simulink model "halogen"  (R2018a)
settings: Solver=ode1  StartTime=0.0  StopTime=11  FixedStep=0.1  RelTol=1e-3
values from neighbouring files (symbols this model uses):
  b = [1/6, 1/3, 1/3, 1/6]    [fensterheber.m]    (also in halogen_script.m = 5; solver_test.m = 1.5e-12)
  Cw = 10    [halogen_script.m]
  k = 3    [halogen_script.m]    (also in solver_test.m = sym('k', [s 1]))
  L = 5    [halogen_script.m]    (also in solver_test.m = 1.5e-05)
  Rc = 10    [halogen_script.m]
  Tu = 30    [halogen_script.m]
settings Model: Creator=Julius  LastModifiedBy=Julius

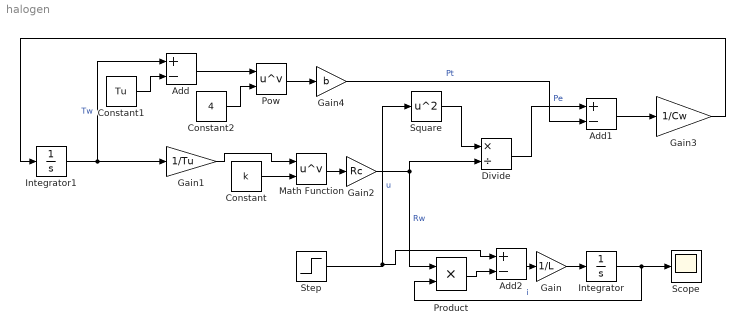
== system halogen ==
  Add : Sum  Inputs=+-
  Add1 : Sum  Inputs=+-
  Add2 : Sum  Inputs=+-
  Constant : Constant  Value=k
  Constant1 : Constant  Value=Tu
  Constant2 : Constant  Value=4
  Divide : Product  Inputs=*/
  Gain : Gain  Gain=1/L
  Gain1 : Gain  Gain=1/Tu
  Gain2 : Gain  Gain=Rc
  Gain3 : Gain  Gain=1/Cw
  Gain4 : Gain  Gain=b
  Integrator : Integrator
  Integrator1 : Integrator  InitialCondition=Tu
  Math Function : Math  Operator=pow  SaturateOnIntegerOverflow=on
  Pow : Math  Operator=pow  RndMeth=Zero  SaturateOnIntegerOverflow=on
  Product : Product  Inputs=**
  Scope : Scope
  Square : Math  Operator=square  SaturateOnIntegerOverflow=on
  Step : Step  SampleTime=0
  wires:
  Integrator/1 -> Product/2, Scope/1  "i"
  Product/1 -> Add2/2
  Step/1 -> Add2/1, Square/1  "u"
  Gain/1 -> Integrator/1
  Math Function/1 -> Gain2/1
  Gain1/1 -> Math Function/1
  Integrator1/1 -> Gain1/1, Add/1  "Tw"
  Constant/1 -> Math Function/2
  Gain2/1 -> Divide/2, Product/1  "Rw"
  Square/1 -> Divide/1
  Divide/1 -> Add1/1  "Pe"
  Constant1/1 -> Add/2
  Add/1 -> Pow/1
  Constant2/1 -> Pow/2
  Pow/1 -> Gain4/1
  Gain4/1 -> Add1/2  "Pt"
  Add1/1 -> Gain3/1
  Gain3/1 -> Integrator1/1
  Add2/1 -> Gain/1
